simulink model "singleRobotControl"  (R2020b)
settings: Solver=VariableStepAuto  StartTime=0.0  StopTime=45  RelTol=1e-3
values from neighbouring files (symbols this model uses):
  loc = zeros(size(p,2), size(p,1))    [map_R.m]    (also in plotter.m)
libraries: mobileRoboticsLib x3, pid_lib x2
settings Model: Creator=Roozbeh  LastModifiedBy=amin1

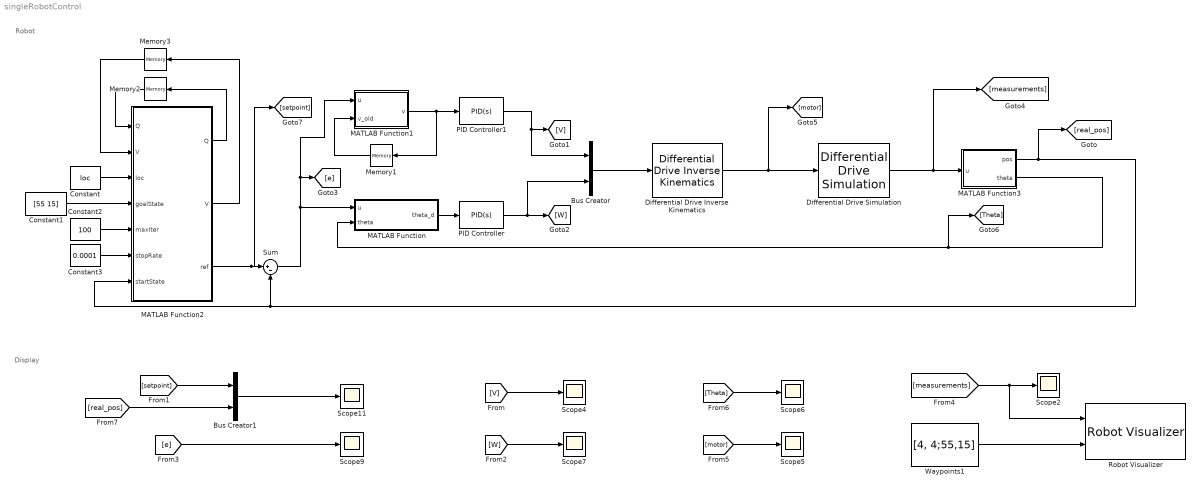
== system singleRobotControl ==
  note: Display
  note: Robot
  Bus Creator : BusCreator  Inputs=2
  Bus Creator1 : BusCreator  Inputs=2
  Constant : Constant  Value=loc
  Constant1 : Constant  Value=[55 15]
  Constant2 : Constant  Value=100
  Constant3 : Constant  Value=0.0001
  Differential Drive Inverse Kinematics : mobileRoboticsLib/Kinematic Models/Differential Drive/Differential Drive Inverse Kinematics  wheelRadius=0.1  wheelBase=0.5
      settings: SourceProductName=Mobile Robotics Simulation Toolbox
  Differential Drive Simulation : mobileRoboticsLib/Kinematic Models/Differential Drive/Differential Drive Simulation  wheelRadius=0.1  wheelBase=0.5  initX=4  initY=4  initAngle=2  Ts=0.05
      settings: SourceProductName=Mobile Robotics Simulation Toolbox
  MATLAB Function : MATLAB Function  TreatAsAtomicUnit=on
  MATLAB Function1 : MATLAB Function  TreatAsAtomicUnit=on
  MATLAB Function2 : MATLAB Function  TreatAsAtomicUnit=on
  MATLAB Function3 : MATLAB Function  TreatAsAtomicUnit=on
  Memory1 : Memory
  Memory2 : Memory  InitialCondition=zeros(size(loc,1) * size(loc,2), 8)
  Memory3 : Memory  InitialCondition=zeros(size(loc,1) * size(loc,2))
  PID Controller : pid_lib/PID Controller  Controller=PID  Form=Parallel  TimeDomain=Continuous-time  UseExternalTs=off  SampleTime=-1  IntegratorMethod=Forward Euler  FilterMethod=Forward Euler  ControllerParametersSource=internal  P=10  I=1  D=0  UseFilter=on  N=100  TunerSelectOption=Transfer Function Based (PID Tuner App)  InitialConditionSource=internal  InitialConditionForIntegrator=0  InitialConditionForFilter=0  DifferentiatorICPrevScaledInput=0  ExternalReset=none  TrackingMode=off  Kt=1  LimitOutput=on  SatLimitsSource=internal  UpperSaturationLimit=5  LowerSaturationLimit=-5  LinearizeAsGain=on  AntiWindupMode=none  Kb=1  POutMin=[]  POutMax=[]  IOutMin=[]  IOutMax=[]  DOutMin=[]  DOutMax=[]  NOutMin=[]  NOutMax=[]  SumOutMin=[]  SumOutMax=[]  SaturationOutMin=[]  SaturationOutMax=[]  PParamMin=[]  PParamMax=[]  IParamMin=[]  IParamMax=[]  DParamMin=[]  DParamMax=[]  NParamMin=[]  NParamMax=[]  KbParamMin=[]  KbParamMax=[]  KtParamMin=[]  KtParamMax=[]  KbOutMin=[]  KbOutMax=[]  KtOutMin=[]  KtOutMax=[]  IntegratorOutMin=[]  IntegratorOutMax=[]  FilterOutMin=[]  FilterOutMax=[]  SumI1OutMin=[]  SumI1OutMax=[]  SumI2OutMin=[]  SumI2OutMax=[]  SumI3OutMin=[]  SumI3OutMax=[]  SumI4OutMin=[]  SumI4OutMax=[]  SumDOutMin=[]  SumDOutMax=[]  DifferentiatorOutMin=[]  DifferentiatorOutMax=[]  FilterDiffOutCoefMin=[]  FilterDiffOutCoefMax=[]  ReciprocalOutMin=[]  ReciprocalOutMax=[]  SumDenOutMin=[]  SumDenOutMax=[]  SumNumOutMin=[]  SumNumOutMax=[]  DivideOutMin=[]  DivideOutMax=[]  UdiffTsProdOutMin=[]  UdiffTsProdOutMax=[]  NTsProdOutMin=[]  NTsProdOutMax=[]  UintegralTsProdOutMin=[]  UintegralTsProdOutMax=[]  UngainTsProdOutMin=[]  UngainTsProdOutMax=[]  IntegratorContinuousStateAttributes=''  IntegratorStateMustResolveToSignalObject=off  IntegratorRTWStateStorageClass=Auto  FilterContinuousStateAttributes=''  FilterStateMustResolveToSignalObject=off  FilterRTWStateStorageClass=Auto  ParallelPVariant=InternalParameters  IdealPVariant=Disabled  IVariant=InternalParameters  DVariant=InternalParameters  IntegratorVariant=Continuous  SatVariant=Enabled  AWVariant=Passthrough  PCopyVariant=Disabled  TRVariant=Disabled  FdbkBlocksVariant=Forward  IdealPFdbkVariant=Disabled  SatFdbkVariant=Disabled  DerivativeFilterVariant=ContFilter  NVariant=InternalParameters  NCopyVariant=Disabled  FilterICVariant=InternalICsFilter  IntegratorICVariant=InternalICs  ExternalResetVariant=Disabled  TRSumVariant=Passthrough  SumFdbkVariant=Disabled  SumVariant=Sum_PID  TsampFilterVariant=InternalTs  TsampNgainVariant=Passthrough  TsampIntegralVariant=Passthrough  ExternalSaturationOutDataTypeStr=Inherit: Same as second input
  PID Controller1 : pid_lib/PID Controller  Controller=PID  Form=Parallel  TimeDomain=Continuous-time  UseExternalTs=off  SampleTime=-1  IntegratorMethod=Forward Euler  FilterMethod=Forward Euler  ControllerParametersSource=internal  P=3  I=0  D=0  UseFilter=on  N=100  TunerSelectOption=Transfer Function Based (PID Tuner App)  InitialConditionSource=internal  InitialConditionForIntegrator=0  InitialConditionForFilter=0  DifferentiatorICPrevScaledInput=0  ExternalReset=none  TrackingMode=off  Kt=1  LimitOutput=on  SatLimitsSource=internal  UpperSaturationLimit=5  LowerSaturationLimit=-5  LinearizeAsGain=on  AntiWindupMode=none  Kb=1  POutMin=[]  POutMax=[]  IOutMin=[]  IOutMax=[]  DOutMin=[]  DOutMax=[]  NOutMin=[]  NOutMax=[]  SumOutMin=[]  SumOutMax=[]  SaturationOutMin=[]  SaturationOutMax=[]  PParamMin=[]  PParamMax=[]  IParamMin=[]  IParamMax=[]  DParamMin=[]  DParamMax=[]  NParamMin=[]  NParamMax=[]  KbParamMin=[]  KbParamMax=[]  KtParamMin=[]  KtParamMax=[]  KbOutMin=[]  KbOutMax=[]  KtOutMin=[]  KtOutMax=[]  IntegratorOutMin=[]  IntegratorOutMax=[]  FilterOutMin=[]  FilterOutMax=[]  SumI1OutMin=[]  SumI1OutMax=[]  SumI2OutMin=[]  SumI2OutMax=[]  SumI3OutMin=[]  SumI3OutMax=[]  SumI4OutMin=[]  SumI4OutMax=[]  SumDOutMin=[]  SumDOutMax=[]  DifferentiatorOutMin=[]  DifferentiatorOutMax=[]  FilterDiffOutCoefMin=[]  FilterDiffOutCoefMax=[]  ReciprocalOutMin=[]  ReciprocalOutMax=[]  SumDenOutMin=[]  SumDenOutMax=[]  SumNumOutMin=[]  SumNumOutMax=[]  DivideOutMin=[]  DivideOutMax=[]  UdiffTsProdOutMin=[]  UdiffTsProdOutMax=[]  NTsProdOutMin=[]  NTsProdOutMax=[]  UintegralTsProdOutMin=[]  UintegralTsProdOutMax=[]  UngainTsProdOutMin=[]  UngainTsProdOutMax=[]  IntegratorContinuousStateAttributes=''  IntegratorStateMustResolveToSignalObject=off  IntegratorRTWStateStorageClass=Auto  FilterContinuousStateAttributes=''  FilterStateMustResolveToSignalObject=off  FilterRTWStateStorageClass=Auto  ParallelPVariant=InternalParameters  IdealPVariant=Disabled  IVariant=InternalParameters  DVariant=InternalParameters  IntegratorVariant=Continuous  SatVariant=Enabled  AWVariant=Passthrough  PCopyVariant=Disabled  TRVariant=Disabled  FdbkBlocksVariant=Forward  IdealPFdbkVariant=Disabled  SatFdbkVariant=Disabled  DerivativeFilterVariant=ContFilter  NVariant=InternalParameters  NCopyVariant=Disabled  FilterICVariant=InternalICsFilter  IntegratorICVariant=InternalICs  ExternalResetVariant=Disabled  TRSumVariant=Passthrough  SumFdbkVariant=Disabled  SumVariant=Sum_PID  TsampFilterVariant=InternalTs  TsampNgainVariant=Passthrough  TsampIntegralVariant=Passthrough  ExternalSaturationOutDataTypeStr=Inherit: Same as second input
  Robot Visualizer : mobileRoboticsLib/Environments/Robot Visualizer  robotRadius=0.7  mapName=mapRooz  showTrajectory=on  hasWaypoints=on  hasLidar=off  sensorOffset=[ 0, 0 ]  scanAngles=[ -pi/4, 0, pi/4 ]  hasObjDetector=off  objDetectorOffset=[ 0, 0 ]  objDetectorAngle=0  objDetectorFOV=pi/4  objDetectorMaxRange=5  objectColors=[ 1, 0, 0; 0, 1, 0; 0, 0, 1 ]
  Scope{2,4..7,9,11} (7 alike) : Scope
  Sum : Sum  Inputs=|+-
  Waypoints1 : Constant  Value=[4, 4;55,15]
  wires:
  Bus Creator/1 -> Differential Drive Inverse Kinematics/1
  PID Controller/1 -> [W], Bus Creator/2
  Sum/1 -> MATLAB Function1/1(u), [e], MATLAB Function/1(u)
  Differential Drive Simulation/1 -> [measurements], MATLAB Function3/1(u)
  Waypoints1/1 -> Robot Visualizer/2
  PID Controller1/1 -> Bus Creator/1, [V]
  MATLAB Function1/1(v) -> Memory1/1, PID Controller1/1
  MATLAB Function/1(theta_d) -> PID Controller/1
  Memory1/1 -> MATLAB Function1/2(v_old)
  MATLAB Function3/2(theta) -> [Theta], MATLAB Function/2(theta)
  Differential Drive Inverse Kinematics/1 -> [motor], Differential Drive Simulation/1
  Bus Creator1/1 -> Scope11/1
  [V] -> Scope4/1
  [W] -> Scope7/1
  [e] -> Scope9/1
  [measurements] -> Scope2/1, Robot Visualizer/1
  [motor] -> Scope5/1
  [Theta] -> Scope6/1
  [real_pos] -> Bus Creator1/2
  [setpoint] -> Bus Creator1/1
  MATLAB Function2/1(Q) -> Memory2/1
  Memory2/1 -> MATLAB Function2/1("Q ")
  MATLAB Function2/2(V) -> Memory3/1
  Memory3/1 -> MATLAB Function2/2("V ")
  Constant/1 -> MATLAB Function2/3(loc)
  Constant1/1 -> MATLAB Function2/4(goalState)
  Constant2/1 -> MATLAB Function2/5(maxIter)
  MATLAB Function3/1(pos) -> Sum/2, MATLAB Function2/7(startState), [real_pos]
  Constant3/1 -> MATLAB Function2/6(stopRate)
  MATLAB Function2/3(ref) -> [setpoint], Sum/1

== matlab function singleRobotControl/MATLAB Function1 ==
  data: u input; v output; v_old input
function v = fcn(u, v_old)

v = sqrt(u(1)^2 + u(2)^2);
if v < 0.3 && v_old < 0.05
    v = 0;
end

== matlab function singleRobotControl/MATLAB Function ==
  data: u input; theta input; theta_d output
function theta_d = fcn(u, theta)

if norm(u) < 0.5
    theta_d = 0;
else
    delta = atan2(u(2), u(1)) - theta;
    sgn = sign(delta);
    delta_hat = delta - 2*pi*sgn;
    if abs(delta_hat) < abs(delta)
        theta_d = delta_hat;
    else
        theta_d = delta;
    end
end

== matlab function singleRobotControl/MATLAB Function2 ==
  data: Q input; Q output; V input; loc input; goalState input; maxIter input; stopRate input; startState input; V output; ref output
function [Q, V, ref] = QLearning(Q, V, loc, goalState, maxIter, stopRate, startState)
    gamma = 0.8;
    alpha = 0.9;
    
    A = [0   1;
         0  -1;
         1   0;
         -1  0;
         1   1;
         1  -1;
         -1  1;
         -1 -1];
    
    numActions = size(A,1);
    m = size(loc,1);
    n = size(loc,2);
    
    Pi = ones(m*n, numActions) / numActions;
    count = 0;
    while count < maxIter
        delta = 0;
        for x = 1:m
            for y = 1:n
                s = (y-1)*m + x;
                v = V(x, y);
                for a = 1:numActions
                    position = [x, y] + A(a,:);
                    R = -norm(A(a,:));
                    %R = -1;
                    if position(1) < 1 || position(1) > m || position(2) < 1 || position(2) > n || loc(round(position(1)), round(position(2))) == 1
                        Q(s, a) = -10;

                    else
                        if position(1) == goalState(1) && position(2) == goalState(2)
                            R = 10;
                        end
                        Q(s, a) = (1 - alpha) * Q(s, a) + alpha*(R + gamma * V(position(1), position(2)));
                    end
                end
                V(x, y) = max(Q(s,:));
                delta = max(delta, abs(v - V(x,y)));
                iter = count;

                Pi(s,:) = Q(s,:) - min(Q(s,:));
                Pi(s,:) = Pi(s,:)/sum(Pi(s,:));
            end
        end
        
        if delta < stopRate
            break;
        end
        count = count + 1;

    end
    
    [~, I] = max(Pi,[],2,'linear');
    Policy = ceil(I/(m*n));
    Policy = reshape(Policy, m, n);
    
    s = round(startState');
    if s(1) == goalState(1) && s(2) == goalState(2)
        ref = s;
    else
        ref = s + A(Policy(s(1),s(2)),:);
    end
end

== matlab function singleRobotControl/MATLAB Function3 ==
  data: u input; pos output; theta output
function [pos, theta] = fcn(u)

pos = u(1:2);
theta = u(3);
